simulink model "AM"  (R2021b)
settings: Solver=VariableStepAuto  StartTime=0.0  StopTime=5  MaxStep=0.00001  RelTol=1e-3
libraries: dsparch4 x1
settings Model: Creator=user  LastModifiedBy=USER

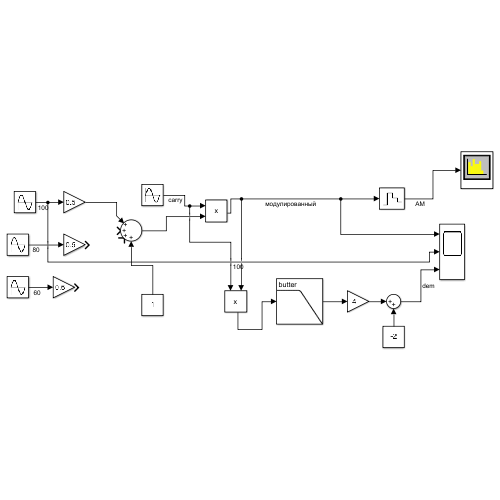
[thumbnail: Simulink's stored preview of the top-level diagram]
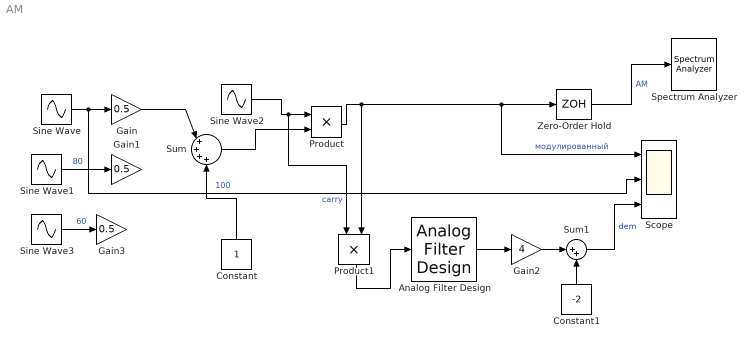
== system AM ==
  Analog Filter Design : dsparch4/Analog Filter Design  method=Butterworth  filttype=Lowpass  N=8  Wlo=1000 * 2 * pi  Whi=80  Rp=2  Rs=40
  Constant : Constant
  Constant1 : Constant  Value=-2
  Gain : Gain  Gain=0.5
  Gain1 : Gain  Gain=0.5
  Gain2 : Gain  Gain=4
  Gain3 : Gain  Gain=0.5
  Product : Product
  Product1 : Product
  Scope : Scope  NumInputPorts=3
  Sine Wave : Sin  Frequency=100 * 2* pi  SampleTime=0
  Sine Wave1 : Sin  Amplitude=1/4  Frequency=80*2*pi  SampleTime=0
  Sine Wave2 : Sin  Frequency=1000 * 2 * pi  SampleTime=0
  Sine Wave3 : Sin  Frequency=2 * pi * 60  SampleTime=0
  Spectrum Analyzer : SpectrumAnalyzer
  Sum : Sum  Inputs=|++++
  Sum1 : Sum  Inputs=|++
  Zero-Order Hold : ZeroOrderHold  SampleTime=1/2500
  wires:
  Sine Wave/1 -> Scope/2, Gain/1  "100"
  Sum/1 -> Product/2
  Constant/1 -> Sum/4
  Sine Wave2/1 -> Product1/1, Product/1  "carry"
  Product/1 -> Scope/1, Zero-Order Hold/1, Product1/2  "модулированный"
  Zero-Order Hold/1 -> Spectrum Analyzer/1  "AM"
  Gain/1 -> Sum/1
  Sine Wave1/1 -> Gain1/1  "80"
  Analog Filter Design/1 -> Gain2/1
  Gain2/1 -> Sum1/1
  Constant1/1 -> Sum1/2
  Product1/1 -> Analog Filter Design/1
  Sine Wave3/1 -> Gain3/1  "60"
  Sum1/1 -> Scope/3  "dem"
